simulink model "hdv_hydroelectropowertrain_model"  (R2026a)
settings: Solver=ode1be  StopTime=simulation_length  FixedStep=tsample  MaxStep=tsample
undefined symbols (not defined in the file): alpha, Apump, available_torque, Bpump, btheta_shaft, C1, consumption, Cpump, dp_lim, E0, E1, E2, E3, E_1, Elog, eta_v_m, eta_v_p, ki_dp_comp, ki_te_comp, kp_ctrl_m, kp_dp_comp, kp_te_comp, Kpump, load_blade_enable, Lpump, M, magnitude, Ncell, Npump, omega_e_rpm_ref, omega_l_max_rpm, q1Kalman, q2Kalman, q3Kalman, Qhr, R0, R1, R_tg, rKalman, rpm_base, rpm_consumption, simulation_length, tau_load, tau_load_max, Tc, torque_base, torque_consumption, torque_friction_base, tsample, v_track1_ref, v_track2_ref, valve_mmorifice_max, xv_m_max
libraries: fl_lib x383, nesl_utility x162, linear_swashplate_ctrl_lib x8, flexshaft_lib x5, bichamber_piston_lib x5, variable_displacement_motor_lib x4, variable_displacement_pump_lib x4, fixed_displacement_pump_lib x4, relief_valve_lib x4, inverse_shuttle_valve_lib x4, hydrostatic_threeway_valve_bichamber_piston_lib x4, hydrostatic_fourway_valve_bichamber_piston_lib x4
(part 5 of 8)

== system hdv_hydroelectropowertrain_model/PR776_powertrain/Hydrostatic_powertrain/driveline_RD2/pressure_charge_system_RD ==
  Hydraulic Flow Rate Sensor : fl_lib/Hydraulic/Hydraulic Sensors/Hydraulic Flow Rate Sensor
  Hydraulic Flow Rate Sensor1 : fl_lib/Hydraulic/Hydraulic Sensors/Hydraulic Flow Rate Sensor
  Hydraulic Pressure Sensor{1..4} (4 alike) : fl_lib/Hydraulic/Hydraulic Sensors/Hydraulic Pressure Sensor
  Hydraulic Reference1 : fl_lib/Hydraulic/Hydraulic Elements/Hydraulic Reference
  Hydraulic Reference2 : fl_lib/Hydraulic/Hydraulic Elements/Hydraulic Reference
  Hydraulic Reference3 : fl_lib/Hydraulic/Hydraulic Elements/Hydraulic Reference
  Mux : Mux  Inputs=2
  PS-Simulink Converter : nesl_utility/PS-Simulink Converter  PhysicalDomain=network_engine_domain  SubClassName=ps_output  LeftPortType=input  RightPortType=output  PseudoPeriodic=off  Frequencies=[]  VectorFormat=1-D array  Unit=l/min  AffineConversion=on
  PS-Simulink Converter{1..3,5} (4 alike) : nesl_utility/PS-Simulink Converter  PhysicalDomain=network_engine_domain  SubClassName=ps_output  LeftPortType=input  RightPortType=output  PseudoPeriodic=off  Frequencies=[]  VectorFormat=1-D array  Unit=bar  AffineConversion=on
  PS-Simulink Converter4 : nesl_utility/PS-Simulink Converter  PhysicalDomain=network_engine_domain  SubClassName=ps_output  LeftPortType=input  RightPortType=output  PseudoPeriodic=off  Frequencies=[]  VectorFormat=1-D array  Unit=l/min  AffineConversion=on
  Scope1 : Scope  NumInputPorts=2
      settings: SampleTime=tsample  ActiveDisplayYMinimum=-11.94319  ActiveDisplayYMaximum=105.50779  DataLoggingVariableName=ScopeData2
  Scope2 : Scope  NumInputPorts=2
      settings: SampleTime=tsample  ActiveDisplayYMinimum=-1.41365  ActiveDisplayYMaximum=12.72285  DataLoggingVariableName=ScopeData2
  Subsystem : Subsystem
  hydro_check_valve1 : Subsystem
      settings: PortSchema="{\"entries\":[{\"content\":{\"sides\":[{\"content\":{\"connectorIds\":[]},\"type\":\"ConnectorPlacement.EquallySpacedRectSide\",\"uuid\":\"a69fbb91-2279-4dfd-af6f-16497d5f1538\"},{\"content\":{\"connectorIds\":[],\"side\":\"RIGHT\"},\"type\":\"ConnectorPlacement.EquallySpacedRectSide\",\"uuid\":\"52e95d44-b7af-4ccc-8556-a2abd2e724e0\"},{\"content\":{\"connectorIds\":[\"LConn1\"],\"side\":\"TOP\"},\"type\":\"ConnectorPlacement.EquallySpacedRectSide\",\"uuid\":\"2d8c071e-4cd0-4b83-8d45-c175cb858754\"},{\"content\":{\"connectorIds\":[\"RConn1\"],\"side\":\"BOTTOM\"},\"type\":\"ConnectorPlacement.EquallySpacedRectSide\",\"uuid\":\"1baec9dc-757c-4f21-904a-6fc08de72ce1\"}]},\"type\":\"ConnectorPlacement.EquallySpacedConnector\",\"uuid\":\"76990e53-6cb0-4bfe-8c9e-427c41b785f2\"}],\"packageUris\":[\"http://schema.mathworks.com/mf0/Connector/19700101\"],\"version\":\"1.0\"}"
  hydro_check_valve2 : Subsystem
      settings: PortSchema="{\"entries\":[{\"content\":{\"sides\":[{\"content\":{\"connectorIds\":[]},\"type\":\"ConnectorPlacement.EquallySpacedRectSide\",\"uuid\":\"a69fbb91-2279-4dfd-af6f-16497d5f1538\"},{\"content\":{\"connectorIds\":[],\"side\":\"RIGHT\"},\"type\":\"ConnectorPlacement.EquallySpacedRectSide\",\"uuid\":\"52e95d44-b7af-4ccc-8556-a2abd2e724e0\"},{\"content\":{\"connectorIds\":[\"LConn1\"],\"side\":\"TOP\"},\"type\":\"ConnectorPlacement.EquallySpacedRectSide\",\"uuid\":\"2d8c071e-4cd0-4b83-8d45-c175cb858754\"},{\"content\":{\"connectorIds\":[\"RConn1\"],\"side\":\"BOTTOM\"},\"type\":\"ConnectorPlacement.EquallySpacedRectSide\",\"uuid\":\"1baec9dc-757c-4f21-904a-6fc08de72ce1\"}]},\"type\":\"ConnectorPlacement.EquallySpacedConnector\",\"uuid\":\"76990e53-6cb0-4bfe-8c9e-427c41b785f2\"}],\"packageUris\":[\"http://schema.mathworks.com/mf0/Connector/19700101\"],\"version\":\"1.0\"}"
  inverse shuttle valve : inverse_shuttle_valve_lib/inverse shuttle valve  pnom=32 bar  dp_crack=0 bar  dp_reg=0 bar  x_rv_max=2 mm  a0=(2*pi*10)^2 1/s^2  a1=2*2*pi*10 1/s  leak=5e-12 m^3/s/Pa  qA_specify=off  qA_priority=None  qA=0 m^3/s  qA_nominal_specify=off  qA_nominal_unit=m^3/s  qA_nominal_value=1  qB_specify=off  qB_priority=None  qB=0 m^3/s  qB_nominal_specify=off  qB_nominal_unit=m^3/s  qB_nominal_value=1  qP_specify=off  qP_priority=None  qP=0 m^3/s  qP_nominal_specify=off  qP_nominal_unit=m^3/s  qP_nominal_value=1  dp_specify=off  dp_priority=None  dp=0 Pa  dp_nominal_specify=off  dp_nominal_unit=Pa  dp_nominal_value=1  dpAP_specify=off  dpAP_priority=None  dpAP=0 Pa  dpAP_nominal_specify=off  dpAP_nominal_unit=Pa  dpAP_nominal_value=1  dpBP_specify=off  dpBP_priority=None  dpBP=0 Pa  dpBP_nominal_specify=off  dpBP_nominal_unit=Pa  dpBP_nominal_value=1  x_rv_AP_specify=off  x_rv_AP_priority=None  x_rv_AP=0 m  x_rv_AP_nominal_specify=off  x_rv_AP_nominal_unit=m  x_rv_AP_nominal_value=1  x_rv_BP_specify=off  x_rv_BP_priority=None  x_rv_BP=0 m  x_rv_BP_nominal_specify=off  x_rv_BP_nominal_unit=m  x_rv_BP_nominal_value=1  x_rv_AP_flt_specify=off  x_rv_AP_flt_priority=None  x_rv_AP_flt=0 m  x_rv_AP_flt_nominal_specify=off  x_rv_AP_flt_nominal_unit=m  x_rv_AP_flt_nominal_value=1  x_rv_BP_flt_specify=off  x_rv_BP_flt_priority=None  x_rv_BP_flt=0 m  x_rv_BP_flt_nominal_specify=off  x_rv_BP_flt_nominal_unit=m  x_rv_BP_flt_nominal_value=1
  qt_ishuttle/dp : Scope  NumInputPorts=2
      settings: SampleTime=tsample  ActiveDisplayYMinimum=-2.35304  ActiveDisplayYMaximum=21.17734
  A : PMIOPort  Side=Left
  B : PMIOPort  Port=2  Side=Right
  D : PMIOPort  Port=3  Side=Right
  wires:
  PS-Simulink Converter5/1 -> qt_ishuttle/dp/2  "dp"
  PS-Simulink Converter4/1 -> qt_ishuttle/dp/1  "qt_ishuttle"
  PS-Simulink Converter3/1 -> Scope2/2  "pCharge"
  PS-Simulink Converter/1 -> Scope2/1, Scope1/2  "qcharge"
  Mux/1 -> Scope1/1
  PS-Simulink Converter1/1 -> Mux/1  "pB"
  PS-Simulink Converter2/1 -> Mux/2  "pA"
  connections:
  inverse shuttle valve/RConn1 -- Hydraulic Flow Rate Sensor1/LConn1
  PS-Simulink Converter5/LConn1 -- Hydraulic Pressure Sensor4/RConn2
  Hydraulic Flow Rate Sensor1/RConn1 -- PS-Simulink Converter4/LConn1
  Hydraulic Flow Rate Sensor1/RConn2 -- Hydraulic Reference3/LConn1
  Hydraulic Reference2/LConn1 -- Hydraulic Pressure Sensor3/RConn1
  Hydraulic Pressure Sensor3/RConn2 -- PS-Simulink Converter3/LConn1
  Subsystem/LConn1 -- D/RConn1
  Hydraulic Flow Rate Sensor/LConn1 -- Subsystem/RConn1 -- Hydraulic Pressure Sensor3/LConn1
  Hydraulic Flow Rate Sensor/RConn1 -- PS-Simulink Converter/LConn1
  Hydraulic Pressure Sensor2/RConn2 -- PS-Simulink Converter2/LConn1
  Hydraulic Pressure Sensor1/RConn2 -- PS-Simulink Converter1/LConn1
  Hydraulic Pressure Sensor1/RConn1 -- Hydraulic Reference1/LConn1 -- Hydraulic Pressure Sensor2/RConn1
  Hydraulic Pressure Sensor1/LConn1 -- hydro_check_valve2/RConn1 -- inverse shuttle valve/LConn2 -- Hydraulic Pressure Sensor4/RConn1 -- B/RConn1
  Hydraulic Pressure Sensor2/LConn1 -- hydro_check_valve1/RConn1 -- inverse shuttle valve/LConn1 -- Hydraulic Pressure Sensor4/LConn1 -- A/RConn1
  hydro_check_valve1/LConn1 -- Hydraulic Flow Rate Sensor/RConn2 -- hydro_check_valve2/LConn1

== system hdv_hydroelectropowertrain_model/PR776_powertrain/Hydrostatic_powertrain/driveline_RD2/vd_ctrl_motor_RD ==
  vd_ref : Inport
  Linear swashplate ctrl2 : linear_swashplate_ctrl_lib/Linear swashplate ctrl  Commented=on  a12=1 1/s  b2=1 1/m/s  k1=100 m  k2=20.5 m  N=5 m  kv=20  xv_specify=off  xv_priority=None  xv=0 m  xv_nominal_specify=off  xv_nominal_unit=m  xv_nominal_value=1  D1_specify=off  D1_priority=None  D1=0  D1_nominal_specify=off  D1_nominal_unit=1  D1_nominal_value=1  D2_specify=off  D2_priority=None  D2=0  D2_nominal_specify=off  D2_nominal_unit=1  D2_nominal_value=1
  PS-Simulink Converter : nesl_utility/PS-Simulink Converter  PhysicalDomain=network_engine_domain  SubClassName=ps_output  LeftPortType=input  RightPortType=output  PseudoPeriodic=off  Frequencies=[]  VectorFormat=1-D array  Unit=inherit  AffineConversion=off
  Scope : Scope  NumInputPorts=2
      settings: ActiveDisplayYMinimum=0.46161  ActiveDisplayYMaximum=1.05982  DataLoggingVariableName=ScopeData2
  Simulink-PS Converter3 : nesl_utility/Simulink-PS Converter  Commented=on  PhysicalDomain=network_engine_domain  SubClassName=ps_input  LeftPortType=input  RightPortType=output  PseudoPeriodic=off  Frequencies=[]  NoiseDistribution=none  NoiseParameters=[]  Unit=1  AffineConversion=off  FilteringAndDerivatives=provide  SimscapeFilterOrder=1  InputFilterTimeConstant=0.001  UdotUserProvided=0
  hose3 : Subsystem
  servo motor LD : Subsystem
  vd : PMIOPort  Side=Right
  pS : PMIOPort  Port=2  Side=Left
  pT : PMIOPort  Port=3  Side=Left
  wires:
  PS-Simulink Converter/1 -> Scope/2
  vd_ref/1 -> servo motor LD/1(displacement reference pu), Simulink-PS Converter3/1, Scope/1
  connections:
  vd/RConn1 -- PS-Simulink Converter/LConn1 -- servo motor LD/RConn1
  Simulink-PS Converter3/RConn1 -- Linear swashplate ctrl2/LConn1
  pT/RConn1 -- hose3/LConn2
  pS/RConn1 -- hose3/LConn1
  hose3/RConn1 -- servo motor LD/LConn1
  hose3/RConn2 -- servo motor LD/LConn2

== system hdv_hydroelectropowertrain_model/PR776_powertrain/Hydrostatic_powertrain/driveline_RD2/vd_ctrl_pump_RD ==
  vd_ref : Inport
  Linear swashplate ctrl2 : linear_swashplate_ctrl_lib/Linear swashplate ctrl  Commented=on  a12=1 1/s  b2=1 1/m/s  k1=100 m  k2=20.5 m  N=5 m  kv=20  xv_specify=off  xv_priority=None  xv=0 m  xv_nominal_specify=off  xv_nominal_unit=m  xv_nominal_value=1  D1_specify=off  D1_priority=None  D1=0  D1_nominal_specify=off  D1_nominal_unit=1  D1_nominal_value=1  D2_specify=off  D2_priority=None  D2=0  D2_nominal_specify=off  D2_nominal_unit=1  D2_nominal_value=1
      settings: InternalSimscapePortConfiguration="{\"Bottom\":[],\"Left\":[{\"id\":\"D_ref\",\"label\":\"Dref\",\"type\":\"input\"}],\"Right\":[{\"id\":\"Dout\",\"label\":\"Dout\",\"type\":\"output\"}],\"Top\":[]}"
  Simulink-PS Converter3 : nesl_utility/Simulink-PS Converter  Commented=on  PhysicalDomain=network_engine_domain  SubClassName=ps_input  LeftPortType=input  RightPortType=output  PseudoPeriodic=off  Frequencies=[]  NoiseDistribution=none  NoiseParameters=[]  Unit=1  AffineConversion=off  FilteringAndDerivatives=provide  SimscapeFilterOrder=1  InputFilterTimeConstant=0.001  UdotUserProvided=0
  hose3 : Subsystem
  servo pump RD : Subsystem
  vd : PMIOPort  Side=Right
  pS : PMIOPort  Port=2  Side=Left
  pT : PMIOPort  Port=3  Side=Left
  wires:
  vd_ref/1 -> Simulink-PS Converter3/1, servo pump RD/1(displacement reference pu)
  connections:
  Simulink-PS Converter3/RConn1 -- Linear swashplate ctrl2/LConn1
  pT/RConn1 -- hose3/LConn2
  pS/RConn1 -- hose3/LConn1
  servo pump RD/LConn1 -- hose3/RConn1
  servo pump RD/LConn2 -- hose3/RConn2
  servo pump RD/RConn1 -- vd/RConn1

== system hdv_hydroelectropowertrain_model/PR776_powertrain/electrical_main_drive_train/LithiumIonBattery/lithium ion cell analytical ocv ==
  Electrical Reference : fl_lib/Electrical/Electrical Elements/Electrical Reference
  PS Constant : fl_lib/Physical Signals/Sources/PS Constant  constant=298.15 K
  PS-Simulink Converter2 : nesl_utility/PS-Simulink Converter  PhysicalDomain=network_engine_domain  SubClassName=ps_output  LeftPortType=input  RightPortType=output  PseudoPeriodic=off  Frequencies=[]  VectorFormat=1-D array  Unit=inherit  AffineConversion=off
  PS-Simulink Converter3 : nesl_utility/PS-Simulink Converter  PhysicalDomain=network_engine_domain  SubClassName=ps_output  LeftPortType=input  RightPortType=output  PseudoPeriodic=off  Frequencies=[]  VectorFormat=1-D array  Unit=inherit  AffineConversion=off
  PS-Simulink Converter4 : nesl_utility/PS-Simulink Converter  PhysicalDomain=network_engine_domain  SubClassName=ps_output  LeftPortType=input  RightPortType=output  PseudoPeriodic=off  Frequencies=[]  VectorFormat=1-D array  Unit=inherit  AffineConversion=off
  lithium-ion battery with analytical OCV : lithium_ion_cell_lib/lithium-ion Cell with analytical OCV  Qcell=Q A*hr  N=Ncell  E_1=E_1 V  E0=E0 V  E1=E1 V  E2=E2 V  E3=E3 V  Elog=Elog V  R0=R0 Ohm  R1=R1 Ohm  C1=C1 F  M=M V  alpha=alpha  u_specify=off  u_priority=High  u=Vdc V  u_nominal_specify=off  u_nominal_unit=V  u_nominal_value=1  u_ocv_specify=off  u_ocv_priority=High  u_ocv=Vdc V  u_ocv_nominal_specify=off  u_ocv_nominal_unit=V  u_ocv_nominal_value=1  icell_specify=on  icell_priority=High  icell=0 A  icell_nominal_specify=off  icell_nominal_unit=A  icell_nominal_value=1  i_r1_specify=off  i_r1_priority=None  i_r1=0 A  i_r1_nominal_specify=off  i_r1_nominal_unit=A  i_r1_nominal_value=1  z_specify=on  z_priority=High  z=soc_init  z_nominal_specify=off  z_nominal_unit=1  z_nominal_value=1  h_specify=off  h_priority=High  h=0  h_nominal_specify=off  h_nominal_unit=1  h_nominal_value=1
  U+ : PMIOPort  Side=Right
  U- : PMIOPort  Port=2  Side=Right
  tag scope: hysteresis=global, icell=global, soc_battery=global
  wires:
  PS-Simulink Converter3/1 -> [soc_battery]  "SOC*"
  PS-Simulink Converter2/1 -> [icell]  "icell"
  PS-Simulink Converter4/1 -> [hysteresis]  "h(t)"
  connections:
  lithium-ion battery with analytical OCV/LConn1 -- PS Constant/RConn1
  lithium-ion battery with analytical OCV/RConn1 -- U+/RConn1
  Electrical Reference/LConn1 -- U-/RConn1 -- lithium-ion battery with analytical OCV/RConn2
  lithium-ion battery with analytical OCV/RConn3 -- PS-Simulink Converter3/LConn1
  lithium-ion battery with analytical OCV/RConn4 -- PS-Simulink Converter2/LConn1
  lithium-ion battery with analytical OCV/RConn5 -- PS-Simulink Converter4/LConn1

== system hdv_hydroelectropowertrain_model/PR776_powertrain/electrical_main_drive_train/dc//dc/iin_ref ==
  current_reference : Subsystem
  iout_ref : Outport
  wires:
  current_reference/1(iin_ref) -> iout_ref/1

== system hdv_hydroelectropowertrain_model/PR776_powertrain/electrical_main_drive_train/dc//dc/iout_ref ==
  current_reference : Subsystem
  iout_ref : Outport
  wires:
  current_reference/1(iout_ref) -> iout_ref/1

== system hdv_hydroelectropowertrain_model/PR776_powertrain/electrical_main_drive_train/dc//dc/sampling_i_filter1 ==
  in : Inport
  1/Ti3 : Gain  Gain=1/150  OutDataTypeStr=double  SaturateOnIntegerOverflow=on  ParamDataTypeStr=Inherit: Same as input
  Saturation : Saturate  UpperLimit=1  LowerLimit=0  OutDataTypeStr=double
  Zero-Order Hold2 : ZeroOrderHold  SampleTime=tsample
  out_pu : Outport
  wires:
  in/1 -> 1/Ti3/1
  1/Ti3/1 -> Saturation/1
  Saturation/1 -> Zero-Order Hold2/1
  Zero-Order Hold2/1 -> out_pu/1

== system hdv_hydroelectropowertrain_model/PR776_powertrain/electrical_main_drive_train/dc//dc/sampling_v_filter1 ==
  in : Inport
  1/Ti3 : Gain  Gain=1/850  OutDataTypeStr=double  SaturateOnIntegerOverflow=on  ParamDataTypeStr=Inherit: Same as input
  Saturation : Saturate  UpperLimit=1  LowerLimit=0  OutDataTypeStr=double
  Zero-Order Hold2 : ZeroOrderHold  SampleTime=tsample
  out_pu : Outport
  wires:
  Zero-Order Hold2/1 -> out_pu/1
  1/Ti3/1 -> Saturation/1
  in/1 -> 1/Ti3/1
  Saturation/1 -> Zero-Order Hold2/1

== system hdv_hydroelectropowertrain_model/PR776_powertrain/electrical_main_drive_train/dc//dc/sampling_v_filter2 ==
  in : Inport
  1/Ti3 : Gain  Gain=1/850  OutDataTypeStr=double  SaturateOnIntegerOverflow=on  ParamDataTypeStr=Inherit: Same as input
  Saturation : Saturate  UpperLimit=1  LowerLimit=0  OutDataTypeStr=double
  Zero-Order Hold2 : ZeroOrderHold  SampleTime=tsample
  out_pu : Outport
  wires:
  in/1 -> 1/Ti3/1
  1/Ti3/1 -> Saturation/1
  Zero-Order Hold2/1 -> out_pu/1
  Saturation/1 -> Zero-Order Hold2/1

== system hdv_hydroelectropowertrain_model/PR776_powertrain/electrical_main_drive_train/dc//dc/sampling_v_filter3 ==
  in : Inport
  1/Ti3 : Gain  Gain=1/150  OutDataTypeStr=double  SaturateOnIntegerOverflow=on  ParamDataTypeStr=Inherit: Same as input
  Saturation : Saturate  UpperLimit=1  LowerLimit=0  OutDataTypeStr=double
  Zero-Order Hold2 : ZeroOrderHold  SampleTime=tsample
  out_pu : Outport
  wires:
  Saturation/1 -> Zero-Order Hold2/1
  Zero-Order Hold2/1 -> out_pu/1
  1/Ti3/1 -> Saturation/1
  in/1 -> 1/Ti3/1

== system hdv_hydroelectropowertrain_model/PR776_powertrain/electrical_main_drive_train/dc//dc/sampling_v_filter4 ==
  in : Inport
  1/Ti3 : Gain  Gain=1/300  OutDataTypeStr=double  SaturateOnIntegerOverflow=on  ParamDataTypeStr=Inherit: Same as input
  Saturation : Saturate  UpperLimit=1  LowerLimit=0  OutDataTypeStr=double
  Zero-Order Hold2 : ZeroOrderHold  SampleTime=tsample
  out_pu : Outport
  wires:
  in/1 -> 1/Ti3/1
  1/Ti3/1 -> Saturation/1
  Zero-Order Hold2/1 -> out_pu/1
  Saturation/1 -> Zero-Order Hold2/1

== system hdv_hydroelectropowertrain_model/PR776_powertrain/electrical_main_drive_train/dc//dc/sampling_v_filter5 ==
  in : Inport
  1/Ti3 : Gain  Gain=1/300  OutDataTypeStr=double  SaturateOnIntegerOverflow=on  ParamDataTypeStr=Inherit: Same as input
  Saturation : Saturate  UpperLimit=1  LowerLimit=0  OutDataTypeStr=double
  Zero-Order Hold2 : ZeroOrderHold  SampleTime=tsample
  out_pu : Outport
  wires:
  Saturation/1 -> Zero-Order Hold2/1
  in/1 -> 1/Ti3/1
  1/Ti3/1 -> Saturation/1
  Zero-Order Hold2/1 -> out_pu/1

== system hdv_hydroelectropowertrain_model/PR776_powertrain/electrical_main_drive_train/dc//dc/vi ctrl ==
  iout : Inport
  vout : Inport  Port=2
  vout_ref : Inport  Port=3
  iout_ref : Inport  Port=4
  iin : Inport  Port=5
  iin_ref : Inport  Port=6
  Iin Ctrl : Subsystem
  Iout Ctrl : Subsystem
  Min : MinMax  Inputs=3
  Sum : Sum  Inputs=++|
  Unit Delay2 : UnitDelay  SampleTime=tsample
  Vout Ctrl : Subsystem
  iin_ref/iin : Scope  NumInputPorts=2
      settings: ActiveDisplayYMinimum=-0.10571  ActiveDisplayYMaximum=0.95137  DataLoggingVariableName=ScopeData7
  iout_ref/iout : Scope  NumInputPorts=2
      settings: ActiveDisplayYMinimum=-0.10571  ActiveDisplayYMaximum=0.95137  DataLoggingVariableName=ScopeData2
  vout_ref/vout : Scope  NumInputPorts=2
      settings: ActiveDisplayYMinimum=-0.10571  ActiveDisplayYMaximum=0.95137  DataLoggingVariableName=ScopeData6
  phase_out : Outport
  wires:
  Unit Delay2/1 -> phase_out/1
  iout/1 -> iout_ref/iout/2, Iout Ctrl/2(iout)
  vout_ref/1 -> vout_ref/vout/1, Vout Ctrl/1(vout_ref)
  vout/1 -> Sum/1, vout_ref/vout/2, Vout Ctrl/2(vout)
  iout_ref/1 -> iout_ref/iout/1, Iout Ctrl/1(iout_ref)
  Iout Ctrl/1(ctrli_out) -> Sum/2
  Sum/1 -> Min/2
  Vout Ctrl/1(ctrlv_out) -> Min/1
  Min/1 -> Unit Delay2/1
  Iin Ctrl/1(ctrli_out) -> Min/3
  iin_ref/1 -> Iin Ctrl/1(iin_ref), iin_ref/iin/1
  iin/1 -> Iin Ctrl/2(iin), iin_ref/iin/2

== system hdv_hydroelectropowertrain_model/PR776_powertrain/electrical_main_drive_train/dc//dc/vout_ref ==
  voltage_reference : Subsystem
  vout_ref : Outport
  wires:
  voltage_reference/1(vout_ref) -> vout_ref/1

== system hdv_hydroelectropowertrain_model/PR776_powertrain/electrical_main_drive_train/pmsm_ctrl/pmsm_dq_ctrl ==
  Bus Creator : BusCreator  Inputs=13
  Capacitor : fl_lib/Electrical/Electrical Elements/Capacitor  c=5e-3 F  r=1e-3 Ohm  g=0 1/Ohm  i_specify=off  i_priority=None  i=0 A  i_nominal_specify=off  i_nominal_value=1  i_nominal_unit=A  v_specify=off  v_priority=High  v=350 V  v_nominal_specify=off  v_nominal_value=1  v_nominal_unit=V  vc_specify=off  vc_priority=High  vc=0 V  vc_nominal_specify=off  vc_nominal_value=1  vc_nominal_unit=V
  Mechanical Rotational Reference : fl_lib/Mechanical/Rotational Elements/Mechanical Rotational Reference
  PS-Simulink Converter1 : nesl_utility/PS-Simulink Converter  PhysicalDomain=network_engine_domain  SubClassName=ps_output  LeftPortType=input  RightPortType=output  PseudoPeriodic=off  Frequencies=[]  VectorFormat=1-D array  Unit=kW  AffineConversion=on
  PS-Simulink Converter10 : nesl_utility/PS-Simulink Converter  PhysicalDomain=network_engine_domain  SubClassName=ps_output  LeftPortType=input  RightPortType=output  PseudoPeriodic=off  Frequencies=[]  VectorFormat=1-D array  Unit=A  AffineConversion=on
  PS-Simulink Converter{2,5,11..13} (5 alike) : nesl_utility/PS-Simulink Converter  PhysicalDomain=network_engine_domain  SubClassName=ps_output  LeftPortType=input  RightPortType=output  PseudoPeriodic=off  Frequencies=[]  VectorFormat=1-D array  Unit=V  AffineConversion=on
  PS-Simulink Converter3 : nesl_utility/PS-Simulink Converter  PhysicalDomain=network_engine_domain  SubClassName=ps_output  LeftPortType=input  RightPortType=output  PseudoPeriodic=off  Frequencies=[]  VectorFormat=1-D array  Unit=A  AffineConversion=on
  PS-Simulink Converter4 : nesl_utility/PS-Simulink Converter  PhysicalDomain=network_engine_domain  SubClassName=ps_output  LeftPortType=input  RightPortType=output  PseudoPeriodic=off  Frequencies=[]  VectorFormat=1-D array  Unit=A  AffineConversion=on
  PS-Simulink Converter6 : nesl_utility/PS-Simulink Converter  PhysicalDomain=network_engine_domain  SubClassName=ps_output  LeftPortType=input  RightPortType=output  PseudoPeriodic=off  Frequencies=[]  VectorFormat=1-D array  Unit=rpm  AffineConversion=on
  PS-Simulink Converter7 : nesl_utility/PS-Simulink Converter  PhysicalDomain=network_engine_domain  SubClassName=ps_output  LeftPortType=input  RightPortType=output  PseudoPeriodic=off  Frequencies=[]  VectorFormat=1-D array  Unit=inherit  AffineConversion=off
  PS-Simulink Converter8 : nesl_utility/PS-Simulink Converter  PhysicalDomain=network_engine_domain  SubClassName=ps_output  LeftPortType=input  RightPortType=output  PseudoPeriodic=off  Frequencies=[]  VectorFormat=1-D array  Unit=inherit  AffineConversion=off
  PS-Simulink Converter9 : nesl_utility/PS-Simulink Converter  PhysicalDomain=network_engine_domain  SubClassName=ps_output  LeftPortType=input  RightPortType=output  PseudoPeriodic=off  Frequencies=[]  VectorFormat=1-D array  Unit=inherit  AffineConversion=off
  Voltage Sensor : fl_lib/Electrical/Electrical Sensors/Voltage Sensor
  phaseU : Subsystem
  pmsm dq controller : pmsm_dq_controller_lib/pmsm dq controller  Speed_mode=simscape.enum.onoff.on  TorqueLim=simscape.enum.onoff.on  emf_nom=ubez V  udc_nom=720.0 V  i_nom=ibez A  omega_m_nom=omega_bez rad/s  poles=poles  Rs=Rs Ohm  Ld=Ld H  Lq=Lq H  phi_m=phi_m V*s  kp_w=kp_w  ki_w=ki_w 1/s  kp_i=kp_i  ki_i=ki_i 1/s  kp_fw=kp_fw  ki_fw=ki_fw 1/s
  pmsm_dq2 : pmsm_dq2_lib/pmsm_dq2  emf_nom=ubez V  i_nom=ibez A  omega_nom=omega_bez rad/s  poles=poles  Rs=Rs Ohm  Ld=Ld H  Lq=Lq H  phi_m=phi_m V*s  J=J kg*m^2  b=b N*m/(rad/s)
  SpeedRef : PMIOPort  Side=Left
  TorqueRef : PMIOPort  Port=2  Side=Left
  D : PMIOPort  Port=3  Side=Right
  Uin+ : PMIOPort  Port=4  Side=Left
  Uin- : PMIOPort  Port=5  Side=Left
  Data : Outport
  wires:
  Bus Creator/1 -> Data/1
  PS-Simulink Converter6/1 -> Bus Creator/1  "speed"
  PS-Simulink Converter7/1 -> Bus Creator/2  "torque"
  PS-Simulink Converter4/1 -> Bus Creator/3  "ig"
  PS-Simulink Converter10/1 -> Bus Creator/4  "id"
  PS-Simulink Converter3/1 -> Bus Creator/5  "iq"
  PS-Simulink Converter8/1 -> Bus Creator/6  "psi_d"
  PS-Simulink Converter9/1 -> Bus Creator/7  "psi_q"
  PS-Simulink Converter5/1 -> Bus Creator/8  "ed"
  PS-Simulink Converter2/1 -> Bus Creator/9  "eq"
  PS-Simulink Converter12/1 -> Bus Creator/10  "vg"
  PS-Simulink Converter11/1 -> Bus Creator/11  "ud"
  PS-Simulink Converter13/1 -> Bus Creator/12  "uq"
  PS-Simulink Converter1/1 -> Bus Creator/13  "pin"
  connections:
  pmsm_dq2/LConn3 -- Mechanical Rotational Reference/LConn1
  pmsm dq controller/RConn1 -- pmsm_dq2/LConn1
  pmsm dq controller/RConn2 -- pmsm_dq2/LConn2
  Capacitor/LConn1 -- Voltage Sensor/LConn1 -- Uin+/RConn1 -- phaseU/LConn2
  phaseU/LConn3 -- Voltage Sensor/RConn2 -- Uin-/RConn1 -- Capacitor/RConn1
  TorqueRef/RConn1 -- pmsm dq controller/LConn8
  SpeedRef/RConn1 -- pmsm dq controller/LConn7
  Voltage Sensor/RConn1 -- pmsm dq controller/LConn6
  D/RConn1 -- pmsm_dq2/RConn14
  pmsm_dq2/RConn1 -- pmsm dq controller/LConn1 -- PS-Simulink Converter6/LConn1
  pmsm_dq2/RConn2 -- PS-Simulink Converter7/LConn1
  pmsm_dq2/RConn3 -- PS-Simulink Converter4/LConn1
  pmsm_dq2/RConn4 -- pmsm dq controller/LConn2 -- PS-Simulink Converter10/LConn1
  pmsm_dq2/RConn5 -- PS-Simulink Converter3/LConn1 -- pmsm dq controller/LConn3
  pmsm_dq2/RConn6 -- PS-Simulink Converter8/LConn1
  pmsm_dq2/RConn7 -- PS-Simulink Converter9/LConn1
  pmsm_dq2/RConn8 -- PS-Simulink Converter5/LConn1 -- pmsm dq controller/LConn4
  pmsm_dq2/RConn9 -- pmsm dq controller/LConn5 -- PS-Simulink Converter2/LConn1
  pmsm_dq2/RConn10 -- PS-Simulink Converter12/LConn1
  PS-Simulink Converter1/LConn1 -- phaseU/LConn1 -- pmsm_dq2/RConn13
  pmsm_dq2/RConn12 -- PS-Simulink Converter13/LConn1
  pmsm_dq2/RConn11 -- PS-Simulink Converter11/LConn1

== system hdv_hydroelectropowertrain_model/PR776_powertrain/front_blade_model/piston_tilt/blade_tilt_model ==
  xp_ref : Inport
  Ideal Force Source : fl_lib/Mechanical/Mechanical Sources/Ideal Force Source
  Ideal Translational Motion Sensor : fl_lib/Mechanical/Mechanical Sensors/Ideal Translational Motion Sensor  reference=foundation.enum.MeasurementReference.difference  acceleration_port=false  velocity_port=true  position_port=true  offset=0 m
  Mass : fl_lib/Mechanical/Translational Elements/Mass  mass=1971.4047 kg  num_ports=foundation.enum.numPorts2.one  v_specify=off  v_priority=High  v=0 m/s  v_nominal_specify=off  v_nominal_value=1  v_nominal_unit=m/s  f_specify=off  f_priority=None  f=0 N  f_nominal_specify=off  f_nominal_value=1  f_nominal_unit=N
  Mechanical Translational Reference1 : fl_lib/Mechanical/Translational Elements/Mechanical Translational Reference
  Mechanical Translational Reference2 : fl_lib/Mechanical/Translational Elements/Mechanical Translational Reference
  PS-Simulink Converter6 : nesl_utility/PS-Simulink Converter  PhysicalDomain=network_engine_domain  SubClassName=ps_output  LeftPortType=input  RightPortType=output  PseudoPeriodic=off  Frequencies=[]  VectorFormat=1-D array  Unit=inherit  AffineConversion=off
  Translational Damper1 : fl_lib/Mechanical/Translational Elements/Translational Damper  D=btheta_shaft N/(m/s)  v_specify=off  v_priority=None  v=0 m/s  v_nominal_specify=off  v_nominal_value=1  v_nominal_unit=m/s  f_specify=off  f_priority=None  f=0 N  f_nominal_specify=off  f_nominal_value=1  f_nominal_unit=N
  Translational Damper4 : fl_lib/Mechanical/Translational Elements/Translational Damper  D=btheta_shaft N/(m/s)  v_specify=off  v_priority=None  v=0 m/s  v_nominal_specify=off  v_nominal_value=1  v_nominal_unit=m/s  f_specify=off  f_priority=None  f=0 N  f_nominal_specify=off  f_nominal_value=1  f_nominal_unit=N
  Translational Spring3 : fl_lib/Mechanical/Translational Elements/Translational Spring  spr_rate=ktheta_shaft N/m  v_specify=off  v_priority=None  v=0 m/s  v_nominal_specify=off  v_nominal_value=1  v_nominal_unit=m/s  f_specify=off  f_priority=None  f=0 N  f_nominal_specify=off  f_nominal_value=1  f_nominal_unit=N  x_specify=off  x_priority=High  x=0 m  x_nominal_specify=off  x_nominal_value=1  x_nominal_unit=m
  xp_re/xp m : Scope  NumInputPorts=2
      settings: ActiveDisplayYMinimum=-0.12375  ActiveDisplayYMaximum=1.11375
  P : PMIOPort  Side=Left
  load : PMIOPort  Port=2  Side=Right
  wires:
  xp_ref/1 -> xp_re/xp m/1
  PS-Simulink Converter6/1 -> xp_re/xp m/2  "xp"
  connections:
  Ideal Force Source/LConn1 -- Ideal Translational Motion Sensor/LConn1 -- Translational Damper4/RConn1 -- Translational Spring3/RConn1 -- Mass/LConn1 -- Translational Damper1/LConn1
  Mechanical Translational Reference2/LConn1 -- Translational Damper1/RConn1
  Translational Damper4/LConn1 -- P/RConn1 -- Translational Spring3/LConn1
  PS-Simulink Converter6/LConn1 -- Ideal Translational Motion Sensor/RConn3
  Ideal Force Source/RConn2 -- Mechanical Translational Reference1/LConn1 -- Ideal Translational Motion Sensor/RConn1
  load/RConn1 -- Ideal Force Source/RConn1

== system hdv_hydroelectropowertrain_model/PR776_powertrain/front_blade_model/piston_tilt/controller ==
  ref : Inport
  xp : Inport  Port=2
  controller : Subsystem
  xv : PMIOPort  Side=Right
  wires:
  ref/1 -> controller/1(ref)
  xp/1 -> controller/2(xp)
  connections:
  xv/RConn1 -- controller/RConn1

== system hdv_hydroelectropowertrain_model/PR776_powertrain/front_blade_model/pistons_height/blade_lift_model ==
  xp_ref : Inport
  Ideal Translational Motion Sensor : fl_lib/Mechanical/Mechanical Sensors/Ideal Translational Motion Sensor  reference=foundation.enum.MeasurementReference.difference  acceleration_port=false  velocity_port=true  position_port=true  offset=0 m
  Mass1 : fl_lib/Mechanical/Translational Elements/Mass  mass=3187.8/3 kg  num_ports=foundation.enum.numPorts2.one  v_specify=off  v_priority=High  v=0 m/s  v_nominal_specify=off  v_nominal_value=1  v_nominal_unit=m/s  f_specify=off  f_priority=None  f=0 N  f_nominal_specify=off  f_nominal_value=1  f_nominal_unit=N
  Mass2 : fl_lib/Mechanical/Translational Elements/Mass  mass=3187.8/3 kg  num_ports=foundation.enum.numPorts2.one  v_specify=off  v_priority=High  v=0 m/s  v_nominal_specify=off  v_nominal_value=1  v_nominal_unit=m/s  f_specify=off  f_priority=None  f=0 N  f_nominal_specify=off  f_nominal_value=1  f_nominal_unit=N
  Mass3 : fl_lib/Mechanical/Translational Elements/Mass  mass=3187.8/3 kg  num_ports=foundation.enum.numPorts2.one  v_specify=off  v_priority=High  v=0 m/s  v_nominal_specify=off  v_nominal_value=1  v_nominal_unit=m/s  f_specify=off  f_priority=None  f=0 N  f_nominal_specify=off  f_nominal_value=1  f_nominal_unit=N
  Mechanical Translational Reference{1..4} (4 alike) : fl_lib/Mechanical/Translational Elements/Mechanical Translational Reference
  PF : fl_lib/Mechanical/Mechanisms/Lever  arm_AC=877.5 mm  arm_BC=877.5 mm  f_A_specify=off  f_A_priority=None  f_A=0 N  f_A_nominal_specify=off  f_A_nominal_value=1  f_A_nominal_unit=N  f_B_specify=off  f_B_priority=None  f_B=0 N  f_B_nominal_specify=off  f_B_nominal_value=1  f_B_nominal_unit=N  f_C_specify=off  f_C_priority=None  f_C=0 N  f_C_nominal_specify=off  f_C_nominal_value=1  f_C_nominal_unit=N
  PS-Simulink Converter15 : nesl_utility/PS-Simulink Converter  PhysicalDomain=network_engine_domain  SubClassName=ps_output  LeftPortType=input  RightPortType=output  PseudoPeriodic=off  Frequencies=[]  VectorFormat=1-D array  Unit=inherit  AffineConversion=off
  Translational Damper{1..7} (7 alike) : fl_lib/Mechanical/Translational Elements/Translational Damper  D=btheta_shaft N/(m/s)  v_specify=off  v_priority=None  v=0 m/s  v_nominal_specify=off  v_nominal_value=1  v_nominal_unit=m/s  f_specify=off  f_priority=None  f=0 N  f_nominal_specify=off  f_nominal_value=1  f_nominal_unit=N
  Translational Spring1 : fl_lib/Mechanical/Translational Elements/Translational Spring  spr_rate=ktheta_shaft N/m  v_specify=off  v_priority=None  v=0 m/s  v_nominal_specify=off  v_nominal_value=1  v_nominal_unit=m/s  f_specify=off  f_priority=None  f=0 N  f_nominal_specify=off  f_nominal_value=1  f_nominal_unit=N  x_specify=off  x_priority=High  x=0 m  x_nominal_specify=off  x_nominal_value=1  x_nominal_unit=m
  Translational Spring2 : fl_lib/Mechanical/Translational Elements/Translational Spring  spr_rate=ktheta_shaft N/m  v_specify=off  v_priority=None  v=0 m/s  v_nominal_specify=off  v_nominal_value=1  v_nominal_unit=m/s  f_specify=off  f_priority=None  f=0 N  f_nominal_specify=off  f_nominal_value=1  f_nominal_unit=N  x_specify=off  x_priority=High  x=0 m  x_nominal_specify=off  x_nominal_value=1  x_nominal_unit=m
  Translational Spring3 : fl_lib/Mechanical/Translational Elements/Translational Spring  spr_rate=ktheta_shaft N/m  v_specify=off  v_priority=None  v=0 m/s  v_nominal_specify=off  v_nominal_value=1  v_nominal_unit=m/s  f_specify=off  f_priority=None  f=0 N  f_nominal_specify=off  f_nominal_value=1  f_nominal_unit=N  x_specify=off  x_priority=High  x=0 m  x_nominal_specify=off  x_nominal_value=1  x_nominal_unit=m
  xp_re/xp m : Scope  NumInputPorts=2
      settings: ActiveDisplayYMinimum=-0.10311  ActiveDisplayYMaximum=0.92803  DataLoggingVariableName=ScopeData3
  PA : PMIOPort  Side=Left
  load : PMIOPort  Port=2  Side=Right
  PB : PMIOPort  Port=3  Side=Left
  wires:
  xp_ref/1 -> xp_re/xp m/1  "xp_ref"
  PS-Simulink Converter15/1 -> xp_re/xp m/2  "xp"
  connections:
  PF/RConn1 -- Translational Spring1/LConn1 -- Translational Damper6/LConn1 -- Translational Damper7/RConn1
  Mechanical Translational Reference3/LConn1 -- Translational Damper3/LConn1
  Mechanical Translational Reference1/LConn1 -- Translational Damper2/LConn1 -- Translational Damper7/LConn1
  Mechanical Translational Reference2/LConn1 -- Translational Damper1/LConn1
  Translational Damper2/RConn1 -- Translational Spring1/RConn1 -- load/RConn1 -- Mass2/LConn1 -- Ideal Translational Motion Sensor/LConn1 -- Translational Damper6/RConn1
  PF/LConn1 -- PA/RConn1 -- Translational Spring3/LConn1 -- Translational Damper4/LConn1
  Translational Spring3/RConn1 -- Translational Damper3/RConn1 -- Mass1/LConn1 -- Translational Damper4/RConn1
  Mass3/LConn1 -- Translational Spring2/RConn1 -- Translational Damper1/RConn1 -- Translational Damper5/RConn1
  Translational Spring2/LConn1 -- PB/RConn1 -- PF/LConn2 -- Translational Damper5/LConn1
  PS-Simulink Converter15/LConn1 -- Ideal Translational Motion Sensor/RConn3
  Ideal Translational Motion Sensor/RConn1 -- Mechanical Translational Reference4/LConn1

== system hdv_hydroelectropowertrain_model/PR776_powertrain/front_blade_model/pistons_height/controller ==
  ref : Inport
  xp : Inport  Port=2
  controller : Subsystem
  xv : PMIOPort  Side=Right
  wires:
  ref/1 -> controller/1(ref)
  xp/1 -> controller/2(xp)
  connections:
  xv/RConn1 -- controller/RConn1

== system hdv_hydroelectropowertrain_model/PR776_powertrain/front_blade_model/pistons_pitch/blade_pitch_model ==
  xpA_ref : Inport
  Blade : fl_lib/Mechanical/Mechanisms/Lever  arm_AC=720 mm  arm_BC=720 mm  f_A_specify=off  f_A_priority=None  f_A=0 N  f_A_nominal_specify=off  f_A_nominal_value=1  f_A_nominal_unit=N  f_B_specify=off  f_B_priority=None  f_B=0 N  f_B_nominal_specify=off  f_B_nominal_value=1  f_B_nominal_unit=N  f_C_specify=off  f_C_priority=None  f_C=0 N  f_C_nominal_specify=off  f_C_nominal_value=1  f_C_nominal_unit=N
  Ideal Translational Motion Sensor : fl_lib/Mechanical/Mechanical Sensors/Ideal Translational Motion Sensor  reference=foundation.enum.MeasurementReference.difference  acceleration_port=false  velocity_port=true  position_port=true  offset=0 m
  Mass : fl_lib/Mechanical/Translational Elements/Mass  mass=1971.4047/2 kg  num_ports=foundation.enum.numPorts2.one  v_specify=off  v_priority=High  v=0 m/s  v_nominal_specify=off  v_nominal_value=1  v_nominal_unit=m/s  f_specify=off  f_priority=None  f=0 N  f_nominal_specify=off  f_nominal_value=1  f_nominal_unit=N
  Mass1 : fl_lib/Mechanical/Translational Elements/Mass  mass=1971.4047/2 kg  num_ports=foundation.enum.numPorts2.one  v_specify=off  v_priority=High  v=0 m/s  v_nominal_specify=off  v_nominal_value=1  v_nominal_unit=m/s  f_specify=off  f_priority=None  f=0 N  f_nominal_specify=off  f_nominal_value=1  f_nominal_unit=N
  Mechanical Translational Reference{1..4} (4 alike) : fl_lib/Mechanical/Translational Elements/Mechanical Translational Reference
  PS-Simulink Converter15 : nesl_utility/PS-Simulink Converter  PhysicalDomain=network_engine_domain  SubClassName=ps_output  LeftPortType=input  RightPortType=output  PseudoPeriodic=off  Frequencies=[]  VectorFormat=1-D array  Unit=inherit  AffineConversion=off
  Translational Damper{1..4} (4 alike) : fl_lib/Mechanical/Translational Elements/Translational Damper  D=btheta_shaft N/(m/s)  v_specify=off  v_priority=None  v=0 m/s  v_nominal_specify=off  v_nominal_value=1  v_nominal_unit=m/s  f_specify=off  f_priority=None  f=0 N  f_nominal_specify=off  f_nominal_value=1  f_nominal_unit=N
  Translational Spring1 : fl_lib/Mechanical/Translational Elements/Translational Spring  spr_rate=ktheta_shaft N/m  v_specify=off  v_priority=None  v=0 m/s  v_nominal_specify=off  v_nominal_value=1  v_nominal_unit=m/s  f_specify=off  f_priority=None  f=0 N  f_nominal_specify=off  f_nominal_value=1  f_nominal_unit=N  x_specify=off  x_priority=High  x=0 m  x_nominal_specify=off  x_nominal_value=1  x_nominal_unit=m
  Translational Spring3 : fl_lib/Mechanical/Translational Elements/Translational Spring  spr_rate=ktheta_shaft N/m  v_specify=off  v_priority=None  v=0 m/s  v_nominal_specify=off  v_nominal_value=1  v_nominal_unit=m/s  f_specify=off  f_priority=None  f=0 N  f_nominal_specify=off  f_nominal_value=1  f_nominal_unit=N  x_specify=off  x_priority=High  x=0 m  x_nominal_specify=off  x_nominal_value=1  x_nominal_unit=m
  xp_re/xp m : Scope  NumInputPorts=2
      settings: ActiveDisplayYMinimum=-0.12375  ActiveDisplayYMaximum=1.11375  DataLoggingVariableName=ScopeData2
  PA : PMIOPort  Side=Left
  PB : PMIOPort  Port=2  Side=Left
  load : PMIOPort  Port=3  Side=Right
  wires:
  PS-Simulink Converter15/1 -> xp_re/xp m/2  "xp"
  xpA_ref/1 -> xp_re/xp m/1
  connections:
  Blade/LConn1 -- PA/RConn1 -- Translational Spring3/LConn1 -- Translational Damper4/LConn1
  Ideal Translational Motion Sensor/RConn1 -- Mechanical Translational Reference4/LConn1
  Blade/LConn2 -- PB/RConn1 -- Translational Damper2/LConn1 -- Translational Spring1/LConn1
  PS-Simulink Converter15/LConn1 -- Ideal Translational Motion Sensor/RConn3
  Blade/RConn1 -- Mechanical Translational Reference2/LConn1
  Ideal Translational Motion Sensor/LConn1 -- Mass/LConn1 -- Translational Damper4/RConn1 -- Translational Damper1/LConn1 -- Translational Spring3/RConn1
  Mechanical Translational Reference3/LConn1 -- Translational Damper1/RConn1
  Mass1/LConn1 -- Translational Spring1/RConn1 -- Translational Damper2/RConn1 -- Translational Damper3/LConn1
  Translational Damper3/RConn1 -- Mechanical Translational Reference1/LConn1

== system hdv_hydroelectropowertrain_model/PR776_powertrain/front_blade_model/pistons_pitch/controller ==
  ref : Inport
  xp : Inport  Port=2
  controller : Subsystem
  xv : PMIOPort  Side=Right
  wires:
  xp/1 -> controller/2(xp)
  ref/1 -> controller/1(ref)
  connections:
  xv/RConn1 -- controller/RConn1

== system hdv_hydroelectropowertrain_model/PR776_powertrain/front_blade_model/pitch_load/pitch_load   ==
  Gain1 : Gain  Gain=load_blade_enable
  Step7 : Step  Time=10  FinalValue=15700  SampleTime=0
  Transfer Fcn : TransferFcn  Denominator=[1e-1 1]
  Out1 : Outport
  wires:
  Gain1/1 -> Transfer Fcn/1
  Step7/1 -> Gain1/1
  Transfer Fcn/1 -> Out1/1

== system hdv_hydroelectropowertrain_model/PR776_powertrain/front_blade_model/tilt_load/tilt_load   ==
  Gain1 : Gain  Gain=load_blade_enable
  Step7 : Step  Time=10  FinalValue=15700  SampleTime=0
  Transfer Fcn : TransferFcn  Denominator=[1e-1 1]
  Out1 : Outport
  wires:
  Step7/1 -> Gain1/1
  Gain1/1 -> Transfer Fcn/1

== system hdv_hydroelectropowertrain_model/PR776_powertrain/front_blade_model/vertical_load/load_disturbance ==
  Gain1 : Gain  Gain=load_blade_enable
  Step7 : Step  Time=10  FinalValue=15700  SampleTime=0
  Transfer Fcn : TransferFcn  Denominator=[1e-1 1]
  Out1 : Outport
  wires:
  Step7/1 -> Gain1/1
  Transfer Fcn/1 -> Out1/1
  Gain1/1 -> Transfer Fcn/1

== system hdv_hydroelectropowertrain_model/Vehicle Control System/synch_overspeed_management/Maximum Speed Control/direction_lineA ==
  In1 : Inport
  Product : Product
  u : Outport
  wires:
  Product/1 -> u/1
  In1/1 -> Product/1
  [direction_SUM] -> Product/2

== system hdv_hydroelectropowertrain_model/PR776_powertrain/Hydrostatic_powertrain/driveine_LD1/pressure_charge_system_LD/Subsystem ==
  Fixed displacement pump : fixed_displacement_pump_lib/Fixed displacement pump  max_Dv=27 cm^3/rev  inertia_pump=0.05 kg*m^2  oil_vol=2.0 l  bp=0.0025 N*m/(rad/s)  lk=1e-6 m  t_specify=off  t_priority=None  t=0 N*m  t_nominal_specify=off  t_nominal_unit=N*m  t_nominal_value=1  q_specify=off  q_priority=None  q=0 m^3/s  q_nominal_specify=off  q_nominal_unit=m^3/s  q_nominal_value=1  qt_specify=off  qt_priority=None  qt=0 m^3/s  qt_nominal_specify=off  qt_nominal_unit=m^3/s  qt_nominal_value=1  qleak_specify=off  qleak_priority=None  qleak=0 m^3/s  qleak_nominal_specify=off  qleak_nominal_unit=m^3/s  qleak_nominal_value=1  Dv_specify=off  Dv_priority=None  Dv=0 cm^3  Dv_nominal_specify=off  Dv_nominal_unit=cm^3  Dv_nominal_value=1  dp_specify=off  dp_priority=None  dp=0 Pa  dp_nominal_specify=off  dp_nominal_unit=Pa  dp_nominal_value=1  we_specify=off  we_priority=None  we=0 rad/s  we_nominal_specify=off  we_nominal_unit=rad/s  we_nominal_value=1
  Hydraulic Reference3 : fl_lib/Hydraulic/Hydraulic Elements/Hydraulic Reference
  Hydraulic Reference4 : fl_lib/Hydraulic/Hydraulic Elements/Hydraulic Reference
  relief valve : relief_valve_lib/relief valve  dp_ref=32 bar  pnom=32 bar  p_set=32 bar  p_reg=12 bar  x_rv_max=12.0 mm  qA_specify=off  qA_priority=None  qA=0 m^3/s  qA_nominal_specify=off  qA_nominal_value=1  qA_nominal_unit=m^3/s  qB_specify=off  qB_priority=None  qB=0 m^3/s  qB_nominal_specify=off  qB_nominal_value=1  qB_nominal_unit=m^3/s  dp_specify=off  dp_priority=None  dp=0 Pa  dp_nominal_specify=off  dp_nominal_value=1  dp_nominal_unit=Pa  x_rv_specify=off  x_rv_priority=None  x_rv=0 m  x_rv_nominal_specify=off  x_rv_nominal_value=1  x_rv_nominal_unit=m  x_rv_flt_specify=off  x_rv_flt_priority=None  x_rv_flt=0 m  x_rv_flt_nominal_specify=off  x_rv_flt_nominal_value=1  x_rv_flt_nominal_unit=m
      settings: LogSimulationData=on
  ps : PMIOPort  Side=Right
  D : PMIOPort  Port=2  Side=Left
  connections:
  Fixed displacement pump/LConn1 -- D/RConn1
  Fixed displacement pump/RConn2 -- Hydraulic Reference3/LConn1
  Hydraulic Reference4/LConn1 -- relief valve/RConn1
  relief valve/LConn1 -- ps/RConn1 -- Fixed displacement pump/RConn1

== system hdv_hydroelectropowertrain_model/PR776_powertrain/Hydrostatic_powertrain/driveine_LD1/pressure_charge_system_LD/hydro_check_valve1 ==
  Constant Area Hydraulic Orifice5 : fl_lib/Hydraulic/Hydraulic Elements/Constant Area Hydraulic Orifice  area=1e-4 mm^2  C_d=1  lam_spec=1  B_lam=0.999  Re_cr=12  q_specify=off  q_priority=None  q=0.001 m^3/s  q_nominal_specify=off  q_nominal_value=1  q_nominal_unit=m^3/s  p_specify=off  p_priority=None  p=0 Pa  p_nominal_specify=off  p_nominal_value=1  p_nominal_unit=Pa
  Constant Area Hydraulic Orifice6 : fl_lib/Hydraulic/Hydraulic Elements/Constant Area Hydraulic Orifice  area=4 mm^2  C_d=1  lam_spec=1  B_lam=0.999  Re_cr=12  q_specify=off  q_priority=None  q=0.001 m^3/s  q_nominal_specify=off  q_nominal_value=1  q_nominal_unit=m^3/s  p_specify=off  p_priority=None  p=0 Pa  p_nominal_specify=off  p_nominal_value=1  p_nominal_unit=Pa
  Hydraulic Flow Rate Sensor : fl_lib/Hydraulic/Hydraulic Sensors/Hydraulic Flow Rate Sensor
  Hydraulic Flow Rate Source : fl_lib/Hydraulic/Hydraulic Sources/Hydraulic Flow Rate Source
  Hydraulic Pressure Sensor : fl_lib/Hydraulic/Hydraulic Sensors/Hydraulic Pressure Sensor
  Hydraulic Pressure Source2 : fl_lib/Hydraulic/Hydraulic Sources/Hydraulic Pressure Source
  Hydraulic Reference : fl_lib/Hydraulic/Hydraulic Elements/Hydraulic Reference
  PS Saturation : fl_lib/Physical Signals/Nonlinear Operators/PS Saturation  upper_limit=inf m^3/s  lower_limit=0 m^3/s  ZeroCross=true
  PS Saturation1 : fl_lib/Physical Signals/Nonlinear Operators/PS Saturation  upper_limit=inf Pa  lower_limit=0 Pa  ZeroCross=true
  PS Transfer Function : fl_lib/Physical Signals/Linear Operators/PS Transfer Function  transfer_function_type=foundation.enum.transfer_function_type.lag  T=tsample s  T1=2 s  T2=1 s  reset_method=foundation.enum.IntegratorResetSpec.None  initial_condition_spec=foundation.enum.IntegratorICSpec.Internal  y0=0 m^3/s
  PS Transfer Function1 : fl_lib/Physical Signals/Linear Operators/PS Transfer Function  transfer_function_type=foundation.enum.transfer_function_type.lag  T=tsample s  T1=2 s  T2=1 s  reset_method=foundation.enum.IntegratorResetSpec.None  initial_condition_spec=foundation.enum.IntegratorICSpec.Internal  y0=0 Pa
  A : PMIOPort  Side=Left
  B : PMIOPort  Port=2  Side=Right
  connections:
  PS Transfer Function/LConn1 -- PS Saturation/RConn1
  PS Saturation1/RConn1 -- PS Transfer Function1/LConn1
  PS Transfer Function/RConn1 -- Hydraulic Flow Rate Source/RConn1
  Constant Area Hydraulic Orifice5/LConn1 -- A/RConn1 -- Hydraulic Pressure Sensor/LConn1 -- Hydraulic Flow Rate Source/RConn2
  Hydraulic Pressure Sensor/RConn2 -- PS Saturation1/LConn1
  PS Transfer Function1/RConn1 -- Hydraulic Pressure Source2/RConn1
  PS Saturation/LConn1 -- Hydraulic Flow Rate Sensor/RConn1
  B/RConn1 -- Constant Area Hydraulic Orifice5/RConn1 -- Hydraulic Pressure Sensor/RConn1 -- Hydraulic Flow Rate Source/LConn1
  Hydraulic Pressure Source2/LConn1 -- Hydraulic Flow Rate Sensor/LConn1
  Hydraulic Pressure Source2/RConn2 -- Hydraulic Reference/LConn1 -- Constant Area Hydraulic Orifice6/RConn1
  Hydraulic Flow Rate Sensor/RConn2 -- Constant Area Hydraulic Orifice6/LConn1

== system hdv_hydroelectropowertrain_model/PR776_powertrain/Hydrostatic_powertrain/driveine_LD1/pressure_charge_system_LD/hydro_check_valve2 ==
  Constant Area Hydraulic Orifice5 : fl_lib/Hydraulic/Hydraulic Elements/Constant Area Hydraulic Orifice  area=1e-4 mm^2  C_d=1  lam_spec=1  B_lam=0.999  Re_cr=12  q_specify=off  q_priority=None  q=0.001 m^3/s  q_nominal_specify=off  q_nominal_value=1  q_nominal_unit=m^3/s  p_specify=off  p_priority=None  p=0 Pa  p_nominal_specify=off  p_nominal_value=1  p_nominal_unit=Pa
  Constant Area Hydraulic Orifice6 : fl_lib/Hydraulic/Hydraulic Elements/Constant Area Hydraulic Orifice  area=4 mm^2  C_d=1  lam_spec=1  B_lam=0.999  Re_cr=12  q_specify=off  q_priority=None  q=0.001 m^3/s  q_nominal_specify=off  q_nominal_value=1  q_nominal_unit=m^3/s  p_specify=off  p_priority=None  p=0 Pa  p_nominal_specify=off  p_nominal_value=1  p_nominal_unit=Pa
  Hydraulic Flow Rate Sensor : fl_lib/Hydraulic/Hydraulic Sensors/Hydraulic Flow Rate Sensor
  Hydraulic Flow Rate Source : fl_lib/Hydraulic/Hydraulic Sources/Hydraulic Flow Rate Source
  Hydraulic Pressure Sensor : fl_lib/Hydraulic/Hydraulic Sensors/Hydraulic Pressure Sensor
  Hydraulic Pressure Source2 : fl_lib/Hydraulic/Hydraulic Sources/Hydraulic Pressure Source
  Hydraulic Reference : fl_lib/Hydraulic/Hydraulic Elements/Hydraulic Reference
  PS Saturation : fl_lib/Physical Signals/Nonlinear Operators/PS Saturation  upper_limit=inf m^3/s  lower_limit=0 m^3/s  ZeroCross=true
  PS Saturation1 : fl_lib/Physical Signals/Nonlinear Operators/PS Saturation  upper_limit=inf Pa  lower_limit=0 Pa  ZeroCross=true
  PS Transfer Function : fl_lib/Physical Signals/Linear Operators/PS Transfer Function  transfer_function_type=foundation.enum.transfer_function_type.lag  T=tsample s  T1=2 s  T2=1 s  reset_method=foundation.enum.IntegratorResetSpec.None  initial_condition_spec=foundation.enum.IntegratorICSpec.Internal  y0=0 m^3/s
  PS Transfer Function1 : fl_lib/Physical Signals/Linear Operators/PS Transfer Function  transfer_function_type=foundation.enum.transfer_function_type.lag  T=tsample s  T1=2 s  T2=1 s  reset_method=foundation.enum.IntegratorResetSpec.None  initial_condition_spec=foundation.enum.IntegratorICSpec.Internal  y0=0 Pa
  A : PMIOPort  Side=Left
  B : PMIOPort  Port=2  Side=Right
  connections:
  Hydraulic Flow Rate Sensor/RConn2 -- Constant Area Hydraulic Orifice6/LConn1
  Constant Area Hydraulic Orifice6/RConn1 -- Hydraulic Reference/LConn1 -- Hydraulic Pressure Source2/RConn2
  Hydraulic Pressure Source2/LConn1 -- Hydraulic Flow Rate Sensor/LConn1
  Hydraulic Flow Rate Source/LConn1 -- Hydraulic Pressure Sensor/RConn1 -- Constant Area Hydraulic Orifice5/RConn1 -- B/RConn1
  PS Saturation/LConn1 -- Hydraulic Flow Rate Sensor/RConn1
  PS Transfer Function1/RConn1 -- Hydraulic Pressure Source2/RConn1
  Hydraulic Pressure Sensor/RConn2 -- PS Saturation1/LConn1
  Hydraulic Flow Rate Source/RConn2 -- Hydraulic Pressure Sensor/LConn1 -- A/RConn1 -- Constant Area Hydraulic Orifice5/LConn1
  PS Transfer Function/RConn1 -- Hydraulic Flow Rate Source/RConn1
  PS Saturation1/RConn1 -- PS Transfer Function1/LConn1
  PS Transfer Function/LConn1 -- PS Saturation/RConn1
